simulink model "Digital_twin_ekf_E3"  (R2025a)
settings: Solver=ode4  StartTime=0.0  StopTime=inf  FixedStep=0.002  RelTol=1e-3  EnableMultiTasking=on
PreLoadFcn:
  | d=fileparts(get_param('Digital_twin_ekf_E3','FileName')); while ~isempty(d)&&~isfile(fullfile(d,'setup_paths.m')), n=fileparts(d); if strcmp(n,d),break;end; d=n; end; if isfile(fullfile(d,'setup_paths.m')), addpath(d); setup_paths; end
  | Ensamblaje_pendulo_furuta_multibody_v4_DataFile;
InitFcn:
  | Ensamblaje_pendulo_furuta_multibody_v4_DataFile;
undefined symbols (not defined in the file): alpha, alphad, int, p, ref, theta, thetad, Vm, xhat
libraries: fl_lib x7, nesl_utility x6, sm_lib x2, simulink_extras x2, ee_lib x1, quarc_library x1, simulink x1
settings Model: ExtModeTrigDuration=10000  Creator=sebas  LastModifiedBy=sebas
settings SolverCC: AlgebraicLoopSolver=TrustRegion  PositivePriorityOrder=on
settings DataIOCC: ReturnWorkspaceOutputs=off
settings DebuggingCC: UnconnectedInputMsg=warning  UnconnectedOutputMsg=warning  UnconnectedLineMsg=warning  ArithmeticOperatorsInVariantConditions=warning
settings ModelReferenceCC: EnableRefExpFcnMdlSchedulingChecks=on
settings SFSimCC: SimUseLocalCustomCode=off  CustomCodeUndefinedFunction=UseInterfaceOnly
settings RTWCC: SystemTargetFile=quarc_win64.tlc  TemplateMakefile=quarc_default_tmf  RTWUseLocalCustomCode=off  Toolchain=QUARC win64 | nmake (64-bit Windows)  BuildConfiguration=Faster Runs  GPUComputeCapability=3.5  Description=QUARC Win64 Target Using Toolchain
settings CodeAppCC: StateflowObjectComments=on
settings STFCustomTargetCC: SystemTargetFile=quarc_win64.tlc  TargetLangStandard=C99 (ISO)  MultiwordLength=2048.0  DynamicStringBufferSize=256.0  ConcurrentExecutionCompliant=on  UseToolchainInfoCompliant=on
settings ConfigComp: CovMetricSettings=dswe
settings ExplorerConfigSet: InternalSimMechanicsExplorerSettings=|
  | <ExplorerConfiguration>
  | 
  |   <canonicalview>planar_xy</canonicalview>
  | 
  |   <TilePanel>
  |     <TileInfo>
  |       <Tiles Columns="1" Count="1" Height="664" Rows="1" Width="1142">
  |         <Row Weight="1"/>
  |         <Column Weight="1"/>
  |         <Tile Height="1" Width="1" X="0" Y="0"/>
  |       </Tiles>
  |     </TileInfo>
  |     <SceneInfo>
  |       <SceneViewer>
  |         <IsThisViewStd>
  |           <IsStandardView>off</IsStandardView>
  |           <StandardViewName>Front</StandardViewName>
  |         </IsThisViewStd>
  |         <BGColor>
  |           <R>1</R>
  |           <G>1</G>
  |           <B>1</B>
  |           <A>1</A>
  |         </BGColor>
  |         <Camera>
  |           <DoPerspective>off</DoPerspective>
  |           <Position>
  |             <X>0.48273089384974083</X>
  |             <Y>0.54863402863013144</Y>
  |             <Z>-0.0083825557684297954</Z>
  |           </Position>
  |           <Center>
  |             <X>-0.015007089263205837</X>
  |             <Y>0.078488323910975918</Y>
  |             <Z>0.036516662315701047</Z>
  |           </Center>
  |           <Up>
  |             <X>-0.5731376381058515</X>
  |             <Y>0.54864415281825929</Y>
  |             <Z>-0.60868944574781358</Z>
  |           </Up>
  |           <XLim>0.11190924142450547</XLim>
  |           <YLim>0.11190924142450547</YLim>
  |           <ViewLimDist>0.01</ViewLimDist>
  |         </Camera>
  |       </SceneViewer>
  |     </SceneInfo>
  |   </TilePanel>
  | 
  |   <MechEditorPanel>
  |     <GfxPanelCameraMap/>
  |     <Cameras/>
  |     <VideoCreator>
  |       <IncludeTiles>All</IncludeTiles>
  |       <IncludeTime>on</IncludeTime>
  |       <IncludeWorldFrame>off</IncludeWorldFrame>
  |       <PlaybackSpeedRatio>1</PlaybackSpeedRatio>
  |       <FrameRate>30</FrameRate>
  |       <FrameSize>auto</FrameSize>
  |       <VideoFormat>UncompressedAVI</VideoFormat>
  |     </VideoCreator>
  |   </MechEditorPanel>
  | 
  |   <PlaybackSettings>
  |     <PlaybackSpeedFactor>1</PlaybackSpeedFactor>
  |   </PlaybackSettings>
  | 
  | </ExplorerConfiguration>

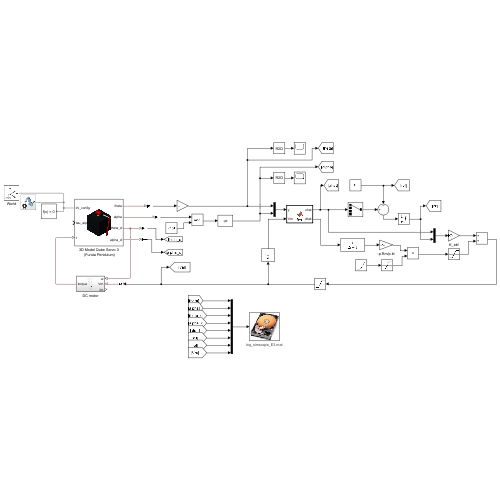
[thumbnail: Simulink's stored preview of the top-level diagram]
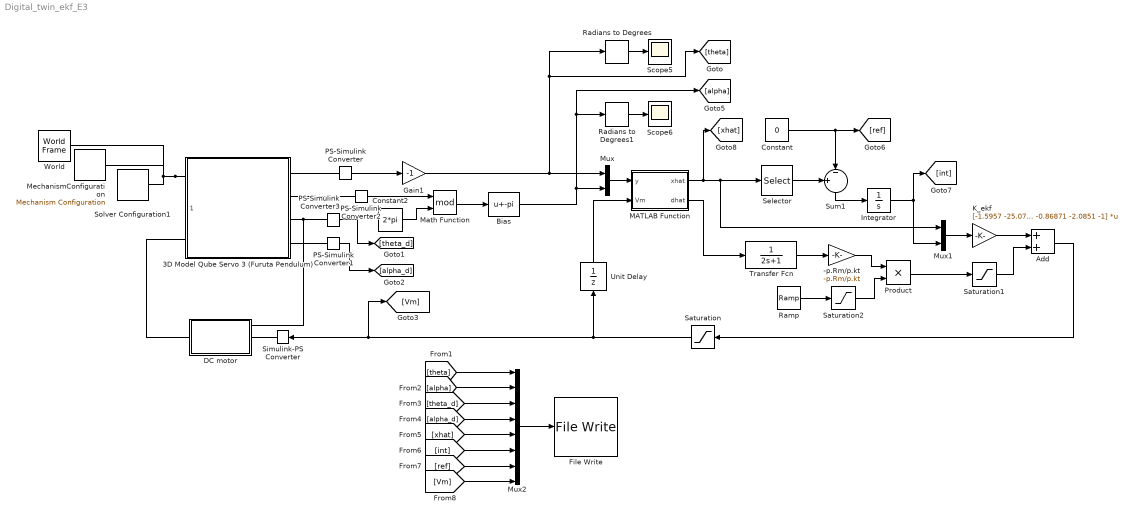
== system Digital_twin_ekf_E3 ==
  -p.Rm/p.kt : Gain  Gain=-p.Rm/p.kt
  3D Model Qube Servo 3 (Furuta Pendulum) : Subsystem  ReferencedSubsystem=Model3d_Furuta_Pendulum
      settings: PortSchema="{\"entries\":[{\"content\":{\"sides\":[{\"content\":{\"connectorIds\":[\"LConn1\",\"In1\",\"RConn1\"]},\"type\":\"ConnectorPlacement.EquallySpacedRectSide\",\"uuid\":\"212e22e8-83aa-4288-bac8-5ec5012ee4e1\"},{\"content\":{\"connectorIds\":[\"RConn2\",\"RConn3\",\"RConn4\",\"RConn5\"],\"side\":\"RIGHT\"},\"type\":\"ConnectorPlacement.EquallySpacedRectSide\",\"uuid\":\"3ce73576-5c91-4b8f-99f3-bf7d5d6df258\"},{\"content\":{\"side\":\"TOP\"},\"type\":\"ConnectorPlacement.EquallySpacedRectSide\",\"uuid\":\"0c3f09e1-5576-45f6-bf17-671c1b7b7e25\"}]},\"type\":\"ConnectorPlacement.EquallySpacedConnector\",\"uuid\":\"8a7c1845-9713-4869-bdf4-33668feaed10\"}],\"packageUris\":[\"http://schema.mathworks.com/mf0/Connector/R2020b\"],\"version\":\"1.0\"}"
  Add : Sum
  Bias : Bias  Bias=-pi  SaturateOnIntegerOverflow=off
  Constant : Constant  Value=0
  Constant2 : Constant  Value=2*pi
  DC motor : Subsystem
  File Write : quarc_library/Sinks/To Target/File Write  source=Specify via dialog (do not evaluate)  file_name=log_simscape_E3.mat  variable_name=theta,alpha,thetad,alphad,xhat,int,ref,Vm  decimation=1  sample_time=-1  file_format=MAT-file v.4  options=No header or footer  append=off  encoding=Default  bitrate=0
      settings: AttributesFormatString=%<file_name>  SourceProductName=QUARC Targets
  Gain1 : Gain  Gain=-1
  Integrator : Integrator  LimitOutput=on  UpperSaturationLimit=2  LowerSaturationLimit=-2
  K_ekf : Gain  Gain=[-1.5957 -25.073 -0.86871 -2.0851 -1]  Multiplication=Matrix(K*u)
  MATLAB Function : MATLAB Function  TreatAsAtomicUnit=on
  Math Function : Math  Operator=mod  SignedPower=on
  MechanismConfiguration : sm_lib/Utilities/Mechanism Configuration  UniformGravity=Constant  GravityVector=[0 -9.7807 0]  GravityVectorUnits=m/s^2  LinearizationDelta=0.001  JointModeTransitionNonlinearIterations=2
  Mux : Mux  Inputs=2
  Mux1 : Mux  Inputs=2
  Mux2 : Mux  Inputs=8
  PS-Simulink Converter{,1..3} (4 alike) : nesl_utility/PS-Simulink Converter  PhysicalDomain=network_engine_domain  SubClassName=ps_output  LeftPortType=input  RightPortType=output  PseudoPeriodic=off  Frequencies=[]  VectorFormat=inherit  Unit=inherit  AffineConversion=off
  Product : Product
  Radians to Degrees : simulink_extras/Transformations/Radians to Degrees
  Radians to Degrees1 : simulink_extras/Transformations/Radians to Degrees
  Ramp : simulink/Sources/Ramp  slope=0.5  start=0  InitialOutput=0
  Saturation : Saturate  UpperLimit=10  LowerLimit=-10
  Saturation1 : Saturate  UpperLimit=2  LowerLimit=-2
  Saturation2 : Saturate  UpperLimit=1  LowerLimit=0
  Scope5 : Scope
      settings: ActiveDisplayYMinimum=-20.612905385229812  ActiveDisplayYMaximum=17.852547514642772  DataLoggingVariableName=ScopeData10
  Scope6 : Scope
      settings: ActiveDisplayYMinimum=-0.30007749157449271  ActiveDisplayYMaximum=0.14537014094803047  DataLoggingVariableName=ScopeData13
  Selector : Selector  InputPortWidth=4  IndexOptions=Index vector (dialog)  Indices=[1]  OutputSizes=1
  Simulink-PS Converter : nesl_utility/Simulink-PS Converter  PhysicalDomain=network_engine_domain  SubClassName=ps_input  LeftPortType=input  RightPortType=output  PseudoPeriodic=off  Frequencies=[]  NoiseDistribution=none  NoiseParameters=[]  Unit=1  AffineConversion=off  FilteringAndDerivatives=filter  SimscapeFilterOrder=1  InputFilterTimeConstant=0.001  UdotUserProvided=0
  Solver Configuration1 : nesl_utility/Solver Configuration  PhysicalDomain=network_engine_domain  SubClassName=solver  LeftPortType=input  RightPortType=generic  Tones=[]  Harmonics=[]  SimulateNoise=off  Profile=off  UseLocalSampling=off  EnableSwitchedLinearOptims=on  FrequencyDomain=off  UseCCode=off  RelTol=0.001  AbsTol=0.001  MinStep=1e-09  ToWorkspace=off  RevertToSquareIcSolve=off  NumHomotopyIterations=100  PhasorMode=off  PhasorModeNumHarmonics=1  ConsistencySolver=NEWTON_XTOL_AFTER_FTOL  IndexReductionMethod=DerivativeReplacement  DoDC=off  ResidualTolerance=1e-09  ConsistencyTolSource=GLOBAL  ConsistencyAbsTol=0.001  ConsistencyRelTol=0.001  ConsistencyTolFactor=1e-9  UseLocalSolver=on  LocalSolverChoice=NE_BACKWARD_EULER_ADVANCER  ResolveIndetEquations=on  FunctionEvalNumThread=1  LocalSolverSampleTime=0.002  DoFixedCost=on  MaxNonlinIter=5  MaxModeIter=2  ComputeImpulses=on  ImpulseIterations=2  LinearAlgebra=auto  LinearAlgebraNumThread=0  EquationFormulation=NE_TIME_EF  DelaysMemoryBudget=1024  AutomaticFiltering=on  FilteringTimeConstant=0.001  PartitionStorageMethod=AS_NEEDED  PartitionMemoryBudget=1024  PartitionMethod=ROBUST  MultibodyUseLocalSolver=off  MultibodyLocalSolverChoice=ODE1  MultibodyLocalSolverSampleTime=0.002
  Sum1 : Sum  Inputs=+|-||
  Transfer Fcn : TransferFcn  Denominator=[2 1]
  Unit Delay : UnitDelay  SampleTime=-1  HasFrameUpgradeWarning=on
  World : sm_lib/Frames and Transforms/World Frame
  wires:
  PS-Simulink Converter/1 -> Gain1/1
  Math Function/1 -> Bias/1
  Constant2/1 -> Math Function/2
  PS-Simulink Converter2/1 -> Math Function/1
  Saturation/1 -> [Vm], Simulink-PS Converter/1, Unit Delay/1
  MATLAB Function/1(xhat) -> [xhat], Mux1/1, Selector/1
  Gain1/1 -> Mux/1, [theta], Radians to Degrees/1
  Bias/1 -> [alpha], Radians to Degrees1/1, Mux/2
  Mux/1 -> MATLAB Function/1(y)
  Radians to Degrees/1 -> Scope5/1
  Radians to Degrees1/1 -> Scope6/1
  K_ekf/1 -> Add/1
  MATLAB Function/2(dhat) -> Transfer Fcn/1
  Transfer Fcn/1 -> -p.Rm/p.kt/1
  -p.Rm/p.kt/1 -> Product/1
  Ramp/1 -> Saturation2/1
  Product/1 -> Saturation1/1
  Saturation1/1 -> Add/2
  Saturation2/1 -> Product/2
  Selector/1 -> Sum1/1
  Constant/1 -> [ref], Sum1/2
  Sum1/1 -> Integrator/1
  Mux1/1 -> K_ekf/1
  Add/1 -> Saturation/1
  Integrator/1 -> [int], Mux1/2
  Unit Delay/1 -> MATLAB Function/2(Vm)
  PS-Simulink Converter3/1 -> [theta_d]
  PS-Simulink Converter1/1 -> [alpha_d]
  Mux2/1 -> File Write/1
  [theta] -> Mux2/1
  [alpha] -> Mux2/2
  [theta_d] -> Mux2/3
  [alpha_d] -> Mux2/4
  [xhat] -> Mux2/5
  [int] -> Mux2/6
  [ref] -> Mux2/7
  [Vm] -> Mux2/8
  connections:
  3D Model Qube Servo 3 (Furuta Pendulum)/LConn1 -- Solver Configuration1/RConn1 -- MechanismConfiguration/RConn1 -- World/RConn1
  Simulink-PS Converter/RConn1 -- DC motor/RConn2
  3D Model Qube Servo 3 (Furuta Pendulum)/RConn1 -- DC motor/LConn1
  3D Model Qube Servo 3 (Furuta Pendulum)/RConn2 -- PS-Simulink Converter/LConn1
  PS-Simulink Converter1/LConn1 -- 3D Model Qube Servo 3 (Furuta Pendulum)/RConn5
  3D Model Qube Servo 3 (Furuta Pendulum)/RConn4 -- DC motor/RConn1 -- PS-Simulink Converter3/LConn1
  3D Model Qube Servo 3 (Furuta Pendulum)/RConn3 -- PS-Simulink Converter2/LConn1

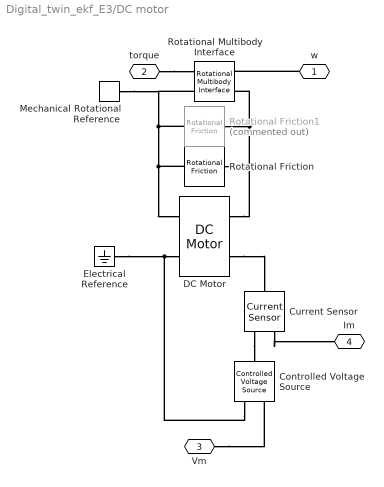
== system Digital_twin_ekf_E3/DC motor ==
  Controlled Voltage Source : fl_lib/Electrical/Electrical Sources/Controlled Voltage Source
  Current Sensor : fl_lib/Electrical/Electrical Sensors/Current Sensor
  DC Motor : ee_lib/Electromechanical/Brushed Motors/DC Motor  field_option=ee.enum.field_option.pm  Rf=100 Ohm  Lf=1 H  Laf=0.15 H  If0=0 A  parameterization=ee.enum.dcparam_option.circuit_param  Ra=7.5 Ohm  La=1.15e-3 H  emf_or_torque=ee.enum.emf_or_torque.kv  Kv=0.0422 V*s/rad  Ki=0.0422 N*m/A  T_stall=0.24e-3 N*m  w_max=5400 rpm  w_rated=4579 rpm  P_rated=9.8 W  V_rated=24 V  lam_param=ee.enum.lam_param.damping  i_noload=16 mA  V_i_noload=24 V  J=1.4e-6 kg*m^2  lam=1*4.8390e-6 N*m*s/rad  speed0=0 rpm  alpha=3.93e-3 1/K  Tmeas=25 degC  thermal_mass=100 J/K  initial_temperature=25 degC
  Electrical Reference : fl_lib/Electrical/Electrical Elements/Electrical Reference
  Mechanical Rotational Reference : fl_lib/Mechanical/Rotational Elements/Mechanical Rotational Reference
  Rotational Friction : fl_lib/Mechanical/Rotational Elements/Rotational Friction  brkwy_trq=1*2.910555e-05+1*4.081637e-05 N*m  brkwy_vel=1.082312e-02 rad/s  Col_trq=2.910555e-05 N*m  visc_coef=4.321929e-06 N*m*s/rad  w_specify=off  w_priority=None  w=0 rad/s  w_nominal_specify=off  w_nominal_value=1  w_nominal_unit=rad/s  t_specify=off  t_priority=None  t=0 N*m  t_nominal_specify=off  t_nominal_value=1  t_nominal_unit=N*m
  Rotational Friction1 : fl_lib/Mechanical/Rotational Elements/Rotational Friction  Commented=on  brkwy_trq=7.066e-04 N*m  brkwy_vel=0.1 rad/s  Col_trq=7.066e-09 N*m  visc_coef=0 N*m*s/rad  w_specify=off  w_priority=None  w=0 rad/s  w_nominal_specify=off  w_nominal_value=1  w_nominal_unit=rad/s  t_specify=off  t_priority=None  t=0 N*m  t_nominal_specify=off  t_nominal_value=1  t_nominal_unit=N*m
  Rotational Multibody Interface : fl_lib/Mechanical/Multibody Interfaces/Rotational Multibody Interface
  w : PMIOPort  Side=Right
  torque : PMIOPort  Port=2  Side=Left
  Vm : PMIOPort  Port=3  Side=Right
  Im : PMIOPort  Port=4  Side=Right
  connections:
  Rotational Friction/LConn1 -- DC Motor/LConn2 -- Rotational Friction1/LConn1 -- Rotational Multibody Interface/RConn2
  torque/RConn1 -- Rotational Multibody Interface/LConn1
  Rotational Friction/RConn1 -- DC Motor/RConn2 -- Rotational Friction1/RConn1 -- Rotational Multibody Interface/LConn2 -- Mechanical Rotational Reference/LConn1
  Vm/RConn1 -- Controlled Voltage Source/RConn1
  w/RConn1 -- Rotational Multibody Interface/RConn1
  DC Motor/RConn1 -- Electrical Reference/LConn1 -- Controlled Voltage Source/RConn2
  Current Sensor/RConn2 -- Controlled Voltage Source/LConn1
  DC Motor/LConn1 -- Current Sensor/LConn1
  Current Sensor/RConn1 -- Im/RConn1

== matlab function Digital_twin_ekf_E3/MATLAB Function ==
  settings: updateMethod=DISCRETE  sampleTime=0.002
  data: y input; xhat output; Vm input; dhat output
function [xhat, dhat] = fcn(y, Vm)
   %#codegen
   [xhat, dhat] = ekf_step(y, Vm);
   end
